simulink model "fourleg_IBC"  (R2022b)
settings: Solver=VariableStepAuto  StartTime=0.0  StopTime=0.2  RelTol=1e-3
libraries: spsCurrentMeasurementLib x10, spsSeriesRLCBranchLib x9, spsDiodeLib x4, spsMosfetLib x4, spsDCVoltageSourceLib x1, spsVoltageMeasurementLib x1, sps_lib x1
settings Model: Creator=vemur  LastModifiedBy=vemur

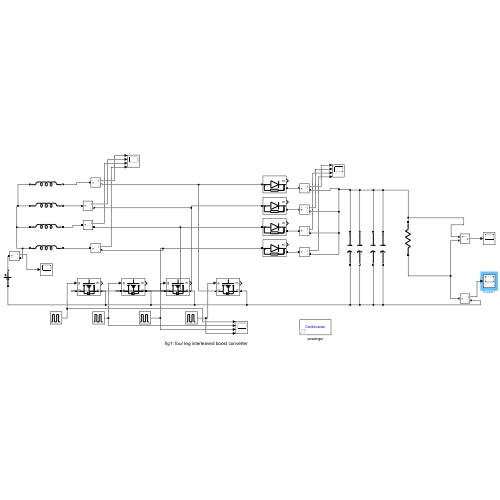
[thumbnail: Simulink's stored preview of the top-level diagram]
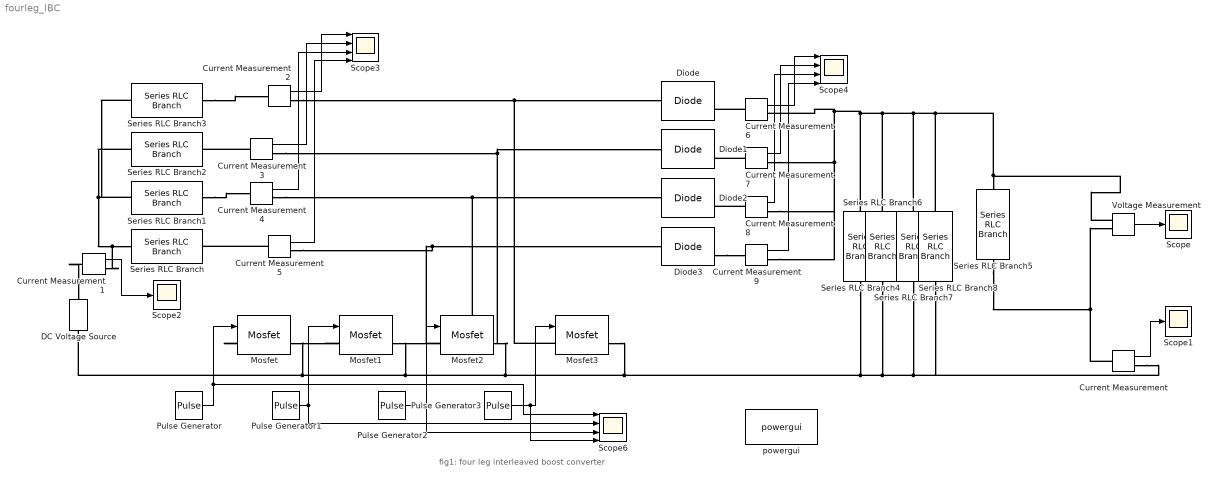
== system fourleg_IBC ==
  note: fig1: four leg interleaved boost converter
  Current Measurement{,1..9} (10 alike) : spsCurrentMeasurementLib/Current Measurement  PhasorSimulation=off  OutputType=Complex  PSBequivalent=0
  DC Voltage Source : spsDCVoltageSourceLib/DC Voltage Source  Amplitude=400  Measurements=None
  Diode{,1..3} (4 alike) : spsDiodeLib/Diode  Ron=0.001  Lon=0  Vf=0.8  IC=0  UseSnubber=0  Rs=500  Cs=250e-9  Measurements=on
  Mosfet{,1..3} (4 alike) : spsMosfetLib/Mosfet  Ron=0.1  Lon=0  Rd=0.01  Vfd=0  IC=0  Rs=1e5  Cs=inf  Measurements=on
  Pulse Generator : DiscretePulseGenerator  PulseType=Time based  Period=1e-4  PulseWidth=50
  Pulse Generator1 : DiscretePulseGenerator  PulseType=Time based  Period=1e-4  PulseWidth=50  PhaseDelay=0.25e-4
  Pulse Generator2 : DiscretePulseGenerator  PulseType=Time based  Period=1e-4  PulseWidth=50  PhaseDelay=0.5e-4
  Pulse Generator3 : DiscretePulseGenerator  PulseType=Time based  Period=1e-4  PulseWidth=50  PhaseDelay=0.75e-4
  Scope : Scope
  Scope1 : Scope
  Scope2 : Scope
  Scope3 : Scope  NumInputPorts=4
  Scope4 : Scope  NumInputPorts=4
  Scope6 : Scope  NumInputPorts=4
  Series RLC Branch{,1..3} (4 alike) : spsSeriesRLCBranchLib/Series RLC Branch  LConnTagsString=__new0  RConnTagsString=__new0  BranchType=L  Resistance=1  Inductance=31.25e-3  SetiL0=off  InitialCurrent=0  Capacitance=1e-6  Setx0=off  InitialVoltage=0  Measurements=None
  Series RLC Branch{4,6..8} (4 alike) : spsSeriesRLCBranchLib/Series RLC Branch  LConnTagsString=__new0  RConnTagsString=__new0  BranchType=C  Resistance=1  Inductance=40e-3  SetiL0=off  InitialCurrent=0  Capacitance=12.5e-6  Setx0=off  InitialVoltage=0  Measurements=None
  Series RLC Branch5 : spsSeriesRLCBranchLib/Series RLC Branch  LConnTagsString=__new0  RConnTagsString=__new0  BranchType=R  Resistance=200  Inductance=40e-3  SetiL0=off  InitialCurrent=0  Capacitance=50e-6  Setx0=off  InitialVoltage=0  Measurements=None
  Voltage Measurement : spsVoltageMeasurementLib/Voltage Measurement  PhasorSimulation=off  OutputType=Complex  PSBequivalent=0
  powergui : sps_lib/powergui  Priority=1  SimulationMode=Continuous  SampleTime=50e-6  frequency=60  Iterations=50  frequencyindice=0  Pbase=100e6  ErrMax=1e-4  UnitsV=kV  UnitsW=MW  buscounter=0  FunctionMessages=off  echomessages=off  EnableUseOfTLC=off  CurrentSourceSwitches=off  DisableSnubberDevices=off  DisableRonSwitches=off  DisableVfSwitches=off  DisplayEquations=off  AutomaticDiscreteSolvers=off  SolverType=Tustin/Backward Euler (TBE)  Interpol=off  ExternalGateDelay=off  methode=off  Ts=100  x0status=blocks  SPID=on  SwTol=0  HookPort=off  NonlinearTolerance=1e-4  nMaxIteration=100  ContinueOnMaxIteration=off  RestoreLinks=warning  ResistiveCurrentMeasurement=off  Frange=[0:2:500]  Ylog=off  Xlog=on  ShowGrid=off  save=off  variable=ZData  structure=0  ZoomFFT=off  StartTime=0.0  cycles=1  DisplayStyle=1  fundamental=60  FreqAxis=off  MaxFrequency=1000  frequencyindicesteady=1  RmsSteady=1  display=off
  wires:
  Pulse Generator/1 -> Scope6/1, Mosfet/1
  Pulse Generator1/1 -> Mosfet1/1, Scope6/2
  Pulse Generator2/1 -> Mosfet2/1, Scope6/3
  Pulse Generator3/1 -> Scope6/4, Mosfet3/1
  Voltage Measurement/1 -> Scope/1
  Current Measurement1/1 -> Scope2/1
  Current Measurement2/1 -> Scope3/1
  Current Measurement3/1 -> Scope3/2
  Current Measurement4/1 -> Scope3/3
  Current Measurement5/1 -> Scope3/4
  Current Measurement6/1 -> Scope4/1
  Current Measurement7/1 -> Scope4/2
  Current Measurement8/1 -> Scope4/3
  Current Measurement9/1 -> Scope4/4
  Current Measurement/1 -> Scope1/1
  connections:
  Series RLC Branch1/LConn1 -- Series RLC Branch3/LConn1 -- Series RLC Branch2/LConn1 -- Current Measurement1/RConn1 -- Series RLC Branch/LConn1
  Mosfet3/LConn1 -- Current Measurement2/RConn1 -- Diode/LConn1
  Mosfet2/LConn1 -- Current Measurement3/RConn1 -- Diode1/LConn1
  Mosfet1/LConn1 -- Current Measurement4/RConn1 -- Diode2/LConn1
  Mosfet/LConn1 -- Current Measurement5/RConn1 -- Diode3/LConn1
  Voltage Measurement/LConn1 -- Series RLC Branch8/LConn1 -- Current Measurement6/RConn1 -- Current Measurement7/RConn1 -- Current Measurement8/RConn1 -- Current Measurement9/RConn1 -- Series RLC Branch4/LConn1 -- Series RLC Branch6/LConn1 -- Series RLC Branch7/LConn1 -- Series RLC Branch5/LConn1
  Series RLC Branch4/RConn1 -- Series RLC Branch8/RConn1 -- Current Measurement/RConn1 -- Series RLC Branch7/RConn1 -- Series RLC Branch6/RConn1 -- Mosfet3/RConn1 -- Mosfet2/RConn1 -- Mosfet/RConn1 -- DC Voltage Source/LConn1 -- Mosfet1/RConn1
  Series RLC Branch5/RConn1 -- Voltage Measurement/LConn2 -- Current Measurement/LConn1
  Current Measurement1/LConn1 -- DC Voltage Source/RConn1
  Series RLC Branch3/RConn1 -- Current Measurement2/LConn1
  Current Measurement3/LConn1 -- Series RLC Branch2/RConn1
  Series RLC Branch1/RConn1 -- Current Measurement4/LConn1
  Current Measurement5/LConn1 -- Series RLC Branch/RConn1
  Current Measurement6/LConn1 -- Diode/RConn1
  Diode3/RConn1 -- Current Measurement9/LConn1
  Current Measurement8/LConn1 -- Diode2/RConn1
  Current Measurement7/LConn1 -- Diode1/RConn1
